simulink model "Multiport_Switch"  (R2014a)
settings: Solver=FixedStepDiscrete  StartTime=0.0  StopTime=10.0  FixedStep=0.1  RelTol=1e-3
settings Model: BufferReuse=off  Creator=kohei-y  LastModifiedBy=ts1413
settings OptimizationCC: BlockReduction=off  OptimizeBlockIOStorage=off  BufferReuse=off  GlobalBufferReuse=off  ExpressionFolding=off  LocalBlockOutputs=off  OptimizeModelRefInitCode=on  LifeSpan=1
settings RTWCC: SystemTargetFile=ert.tlc  GenCodeOnly=on  TemplateMakefile=ert_default_tmf  Description=Embedded Coder  ProcessScript=ert_make_rtw_hook  IncludeHyperlinkInReport=on
settings CodeAppCC: IgnoreCustomStorageClasses=off
settings ERTTargetCC: ParMdlRefBuildCompliant=on  CompOptLevelCompliant=on  ConcurrentExecutionCompliant=on  ERTFirstTimeCompliant=on  ModelStepFunctionPrototypeControlCompliant=on  CPPClassGenCompliant=on  InlinedParameterPlacement=Hierarchical  ERTCustomFileTemplate=example_file_process.tlc

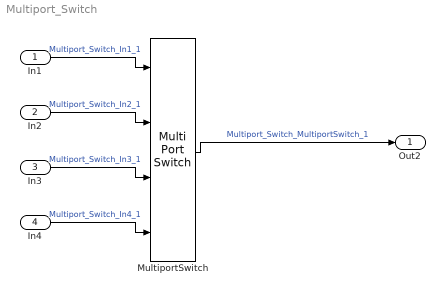
== system Multiport_Switch ==
  In1 : Inport
  In2 : Inport  Port=2
  In3 : Inport  Port=3
  In4 : Inport  Port=4
  MultiportSwitch : MultiPortSwitch  DiagnosticForDefault=None
  Out2 : Outport
  wires:
  In1/1 -> MultiportSwitch/1  "Multiport_Switch_In1_1"
  In2/1 -> MultiportSwitch/2  "Multiport_Switch_In2_1"
  In4/1 -> MultiportSwitch/4  "Multiport_Switch_In4_1"
  In3/1 -> MultiportSwitch/3  "Multiport_Switch_In3_1"
  MultiportSwitch/1 -> Out2/1  "Multiport_Switch_MultiportSwitch_1"
